simulink model "MECN4029-Group15-Solar-Tracker"  (R2024a)
settings: Solver=ode5  StartTime=0.0  StopTime=400  FixedStep=0.01  RelTol=1e-3
libraries: simulink_extras x5

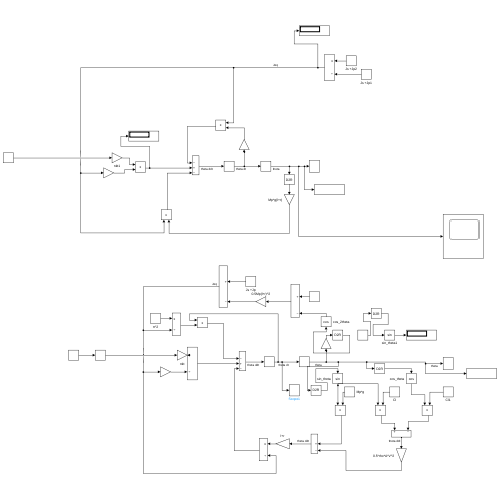
[thumbnail: Simulink's stored preview of the top-level diagram]
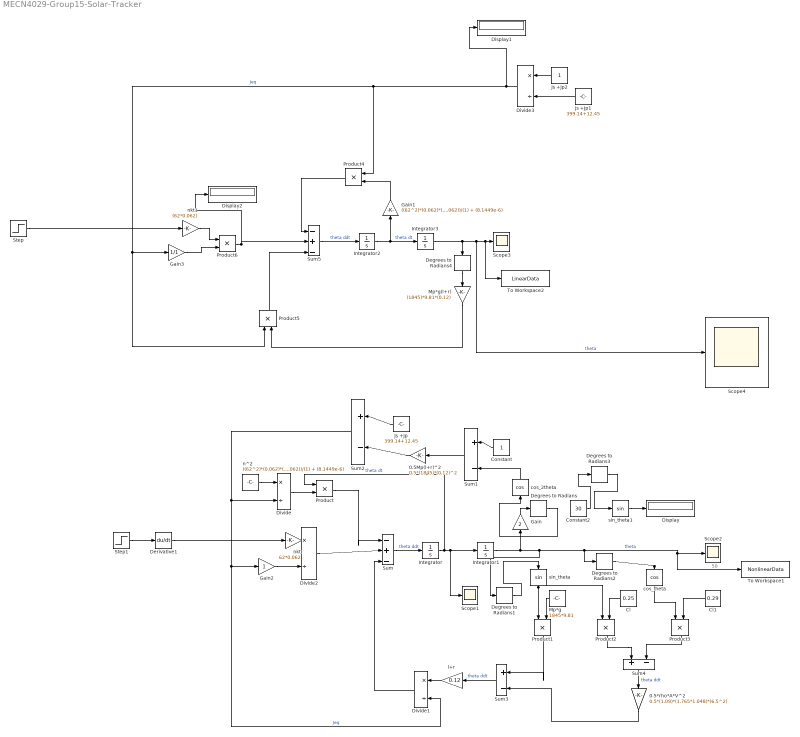
== system MECN4029-Group15-Solar-Tracker ==
  note: 50
  0.5*rho*A*V^2 : Gain  Gain=0.5*(1.09)*(1.765*1.048)*(6.5^2)
  0.5Mp(l+r)^2 : Gain  Gain=0.5*(1845)*(0.12)^2
  Cl : Constant  Value=0.25
  Cl1 : Constant  Value=0.29
  Constant : Constant
  Constant2 : Constant  Value=30
  Degrees to Radians{,1..4} (5 alike) : simulink_extras/Transformations/Degrees to Radians
  Derivative1 : Derivative
  Display : Display
  Display1 : Display
  Display2 : Display
  Divide{,1..3} (4 alike) : Product  Inputs=*/
  Gain : Gain  Gain=2
  Gain1 : Gain  Gain=((62^2)*(0.062)*(0.062))/(1) + (8.1449e-6)
  Gain2 : Gain
  Gain3 : Gain  Gain=1/1
  Integrator{,1..3} (4 alike) : Integrator
  Js +Jp : Constant  Value=399.14+12.45
  Js +Jp1 : Constant  Value=399.14+12.45
  Js +Jp2 : Constant
  Mp*g : Constant  Value=1845*9.81
  Mp*g(l+r) : Gain  Gain=(1845)*9.81*(0.12)
  Product{,1..6} (7 alike) : Product
  Scope{1..4} (4 alike) : Scope
  Step : Step  Time=0  After=24  SampleTime=0
  Step1 : Step  Time=0.05  After=24  SampleTime=0
  Sum : Sum  Inputs=|-+-
  Sum1 : Sum  Inputs=|+|-
  Sum2 : Sum  Inputs=|+|-
  Sum3 : Sum  Inputs=|+-
  Sum4 : Sum  Inputs=+|-
  Sum5 : Sum  Inputs=|-+-
  To Workspace1 : ToWorkspace  VariableName=NonlinearData  SaveFormat=Timeseries  SampleTime=-1
      settings: Save2DSignal=2-D array (concatenate along first dimension)
  To Workspace2 : ToWorkspace  VariableName=LinearData  SaveFormat=Timeseries  SampleTime=-1
      settings: Save2DSignal=2-D array (concatenate along first dimension)
  cos_2theta : Trigonometry  Operator=cos
  cos_theta : Trigonometry  Operator=cos
  l+r : Gain  Gain=0.12
  n^2 : Constant  Value=((62^2)*(0.062)*(0.062))/(1) + (8.1449e-6)
  nkt : Gain  Gain=62*0.062
  nkt1 : Gain  Gain=(62*0.062)
  sin_theta : Trigonometry
  sin_theta1 : Trigonometry
  wires:
  Sum/1 -> Integrator/1  "theta ddt"
  Integrator/1 -> Integrator1/1, Scope1/1, Product/1  "theta dt"
  Integrator1/1 -> Gain/1, Degrees to Radians1/1, Scope2/1, To Workspace1/1, Degrees to Radians2/1  "theta"
  Gain/1 -> Degrees to Radians/1
  cos_2theta/1 -> Sum1/2
  Constant/1 -> Sum1/1
  Sum1/1 -> 0.5Mp(l+r)^2/1
  0.5Mp(l+r)^2/1 -> Sum2/2
  Js +Jp/1 -> Sum2/1
  Sum2/1 -> Divide1/2, Gain2/1, Divide/2  "Jeq"
  n^2/1 -> Divide/1
  Divide/1 -> Product/2
  Product/1 -> Sum/1
  sin_theta/1 -> Product2/1, Product1/1
  Mp*g/1 -> Product1/2
  Cl/1 -> Product2/2
  cos_theta/1 -> Product3/1
  Cl1/1 -> Product3/2
  Product1/1 -> Sum3/1
  Product3/1 -> Sum4/2
  Product2/1 -> Sum4/1
  Sum4/1 -> 0.5*rho*A*V^2/1  "theta ddt"
  0.5*rho*A*V^2/1 -> Sum3/2
  Sum3/1 -> l+r/1  "theta ddt"
  l+r/1 -> Divide1/1
  Divide1/1 -> Sum/3
  nkt/1 -> Divide2/1
  Divide2/1 -> Sum/2
  Gain2/1 -> Divide2/2
  Constant2/1 -> Degrees to Radians3/1
  sin_theta1/1 -> Display/1
  Degrees to Radians/1 -> cos_2theta/1
  Degrees to Radians1/1 -> sin_theta/1
  Degrees to Radians2/1 -> cos_theta/1
  Degrees to Radians3/1 -> sin_theta1/1
  Sum5/1 -> Integrator2/1  "theta ddt"
  Integrator2/1 -> Integrator3/1, Gain1/1  "theta dt"
  Integrator3/1 -> To Workspace2/1, Scope3/1, Scope4/1, Degrees to Radians4/1  "theta"
  Js +Jp1/1 -> Divide3/2
  Js +Jp2/1 -> Divide3/1
  Gain1/1 -> Product4/2
  Divide3/1 -> Display1/1, Product5/1, Gain3/1, Product4/1  "Jeq"
  Product4/1 -> Sum5/1
  Mp*g(l+r)/1 -> Product5/2
  Product5/1 -> Sum5/3
  Gain3/1 -> Product6/2
  Product6/1 -> Display2/1, Sum5/2
  nkt1/1 -> Product6/1
  Degrees to Radians4/1 -> Mp*g(l+r)/1
  Derivative1/1 -> nkt/1
  Step/1 -> nkt1/1
  Step1/1 -> Derivative1/1
